simulink model "PV_battery"  (R2020a)
settings: Solver=FixedStepDiscrete  StartTime=0.0  StopTime=20  FixedStep=Tss  RelTol=1e-3
values from neighbouring files (symbols this model uses):
  Ccbattery = 1000e-6    (= 0.001)    [pv_battery.m]
  Ccboost = 3300e-6    (= 0.0033)    [pv_battery.m]
  Ccpv = 100e-6    (= 0.0001)    [pv_battery.m]
  DB_max = 0.95    [pv_battery.m]
  DB_min = 0    [pv_battery.m]
  Delta = 125e-6    (= 0.000125)    [pv_battery.m]
  I_discharge = 22    [pv_battery.m]
  Ki_B1 = 10    [pv_battery.m]
  Ki_B2 = 10    [pv_battery.m]
  Kp_B1 = 0.01    [pv_battery.m]
  Kp_B2 = 0.85    [pv_battery.m]
  LL = 5e-3    (= 0.005)    [pv_battery.m]
  LL1 = 0.5e-3    (= 0.0005)    [pv_battery.m]
  Rcbattery = 1e-4    (= 0.0001)    [pv_battery.m]
  Rcboost = 1e-4    (= 0.0001)    [pv_battery.m]
  Rcpv = 1e-4    (= 0.0001)    [pv_battery.m]
  RL = 0.1    [pv_battery.m]
  RL1 = 0.1    [pv_battery.m]
  Tss = 10e-6    (= 1e-05)    [pv_battery.m]
  Tsspid1 = 5*Tss    (= 5e-05)    [pv_battery.m]
  Tsspid2 = 50*Tss    (= 0.0005)    [pv_battery.m]
  v_bus_ref = 48    [pv_battery.m]
undefined symbols (not defined in the file or in its folder): Ion, Lithium
libraries: powerlib x13, simulink x2, powerlib_meascontrol x2, electricdrivelib x1, re_lib x1
settings Model: Creator=Junaed  LastModifiedBy=Junaed

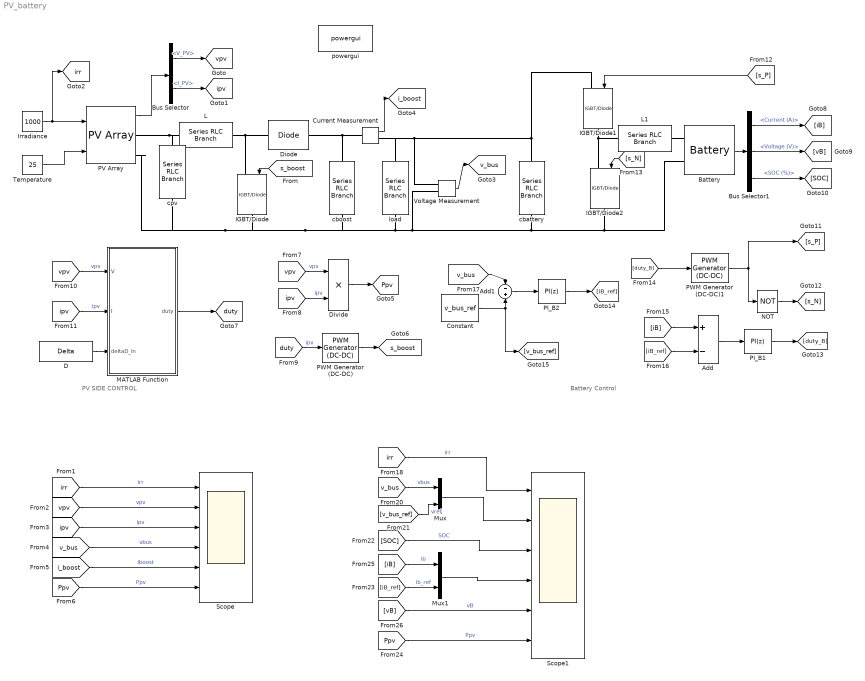
== system PV_battery ==
  note: PV SIDE CONTROL
  note: Battery Control
  Add : Sum  Inputs=+-
  Add1 : Sum  Inputs=-+
  Battery : electricdrivelib/Extra Sources/Battery  BatType=Lithium-Ion  ShowTempParam=off  ThermalPreset=no  ShowAgeParam=off  NomV=Vbat_nom  NomQ=Capacity_nom  SOC=SOC_in  Batt_Tr=1  PresetModel=on  MaxQ=50  MinV=18  FullV=27.9357  Dis_rate=21.7391  R=0.0048  Normal_OP=45.2174  expZone="[25.9293      2.45652]"  current=[6.5 13 32.5]  Units=Time  Tci=20  NomT=20  T2=-30  MaxQ2=4.8  FullV2=7.1  Normal_OP2=5.655  expZone2="[6.58           1]"  Rca=0.6  ti=2000  Dp=0  Neq0=0  Tsim=1e6  Ta1=25  Qeol=5.4*0.9  Reol=0.013333*1.2  Char_age=[2.3478, 3]  Dis_age=[2.3478, 10]  N1=1500  N2=10500  N3=1000  N4=1400  Ta2=45  N5=950
  Bus Selector : BusSelector  OutputSignals=V_PV,I_PV
  Bus Selector1 : BusSelector  OutputSignals=Current (A),Voltage (V),SOC (%)
  Constant : Constant  Value=v_bus_ref
  Current Measurement : powerlib/Measurements/Current Measurement  PhasorSimulation=off  OutputType=Complex  PSBequivalent=0
  D : Constant  Value=Delta
  Diode : powerlib/Power Electronics/Diode  Ron=0.001  Lon=0  Vf=0.8  IC=0  UseSnubber=0  Rs=500  Cs=250e-9  Measurements=off
  Divide : Product  Inputs=**
  IGBT/Diode : powerlib/Power Electronics/IGBT//Diode  Ron=1e-3  Rs=1e5  Cs=inf  Measurements=off
  IGBT/Diode1 : powerlib/Power Electronics/IGBT//Diode  Ron=1e-3  Rs=1e5  Cs=inf  Measurements=off
  IGBT/Diode2 : powerlib/Power Electronics/IGBT//Diode  Ron=1e-3  Rs=1e5  Cs=inf  Measurements=off
  Irradiance : Constant  Value=1000
  L : powerlib/Elements/Series RLC Branch  LConnTagsString=__new0  RConnTagsString=__new0  BranchType=RL  Resistance=RL  Inductance=LL  SetiL0=off  InitialCurrent=0  Capacitance=100e-6  Setx0=off  InitialVoltage=0  Measurements=None
  L1 : powerlib/Elements/Series RLC Branch  LConnTagsString=__new0  RConnTagsString=__new0  BranchType=RL  Resistance=RL1  Inductance=LL1  SetiL0=off  InitialCurrent=0  Capacitance=100e-6  Setx0=off  InitialVoltage=0  Measurements=None
  MATLAB Function : MATLAB Function  TreatAsAtomicUnit=on
  Mux : Mux  Inputs=2
  Mux1 : Mux  Inputs=2
  NOT : Logic  Operator=NOT  IconShape=distinctive  AllPortsSameDT=off  OutDataTypeStr=boolean
  PI_B1 : simulink/Continuous/PID Controller  Controller=PI  Form=Parallel  TimeDomain=Discrete-time  UseExternalTs=off  SampleTime=Tsspid1  IntegratorMethod=Forward Euler  FilterMethod=Forward Euler  ControllerParametersSource=internal  P=Kp_B1  I=Ki_B1  D=0  UseFilter=on  N=100  TunerSelectOption=Transfer Function Based (PID Tuner App)  InitialConditionSource=internal  InitialConditionForIntegrator=0  InitialConditionForFilter=0  DifferentiatorICPrevScaledInput=0  ExternalReset=none  TrackingMode=off  Kt=1  LimitOutput=on  UpperSaturationLimit=DB_max  LowerSaturationLimit=DB_min  LinearizeAsGain=off  AntiWindupMode=none  Kb=1  POutMin=[]  POutMax=[]  IOutMin=[]  IOutMax=[]  DOutMin=[]  DOutMax=[]  NOutMin=[]  NOutMax=[]  SumOutMin=[]  SumOutMax=[]  SaturationOutMin=[]  SaturationOutMax=[]  PParamMin=[]  PParamMax=[]  IParamMin=[]  IParamMax=[]  DParamMin=[]  DParamMax=[]  NParamMin=[]  NParamMax=[]  KbParamMin=[]  KbParamMax=[]  KtParamMin=[]  KtParamMax=[]  KbOutMin=[]  KbOutMax=[]  KtOutMin=[]  KtOutMax=[]  IntegratorOutMin=[]  IntegratorOutMax=[]  FilterOutMin=[]  FilterOutMax=[]  SumI1OutMin=[]  SumI1OutMax=[]  SumI2OutMin=[]  SumI2OutMax=[]  SumI3OutMin=[]  SumI3OutMax=[]  SumI4OutMin=[]  SumI4OutMax=[]  SumDOutMin=[]  SumDOutMax=[]  DifferentiatorOutMin=[]  DifferentiatorOutMax=[]  FilterDiffOutCoefMin=[]  FilterDiffOutCoefMax=[]  ReciprocalOutMin=[]  ReciprocalOutMax=[]  SumDenOutMin=[]  SumDenOutMax=[]  SumNumOutMin=[]  SumNumOutMax=[]  DivideOutMin=[]  DivideOutMax=[]  UdiffTsProdOutMin=[]  UdiffTsProdOutMax=[]  NTsProdOutMin=[]  NTsProdOutMax=[]  UintegralTsProdOutMin=[]  UintegralTsProdOutMax=[]  UngainTsProdOutMin=[]  UngainTsProdOutMax=[]  IntegratorContinuousStateAttributes=''  IntegratorStateMustResolveToSignalObject=off  IntegratorRTWStateStorageClass=Auto  FilterContinuousStateAttributes=''  FilterStateMustResolveToSignalObject=off  FilterRTWStateStorageClass=Auto  ParallelPVariant=InternalParameters  IdealPVariant=Disabled  IVariant=InternalParameters  DVariant=Disabled  IntegratorVariant=Discrete  SatVariant=Enabled  AWVariant=Passthrough  PCopyVariant=Disabled  TRVariant=Disabled  FdbkBlocksVariant=Forward  IdealPFdbkVariant=Disabled  SatFdbkVariant=Disabled  DerivativeFilterVariant=Disabled  NVariant=Disabled  NCopyVariant=Disabled_SignalSpec  FilterICVariant=Disabled  IntegratorICVariant=InternalICs  ExternalResetVariant=Disabled  TRSumVariant=Passthrough  SumFdbkVariant=Disabled  SumVariant=Sum_PI  TsampFilterVariant=InternalTs  TsampNgainVariant=Passthrough  TsampIntegralVariant=Passthrough
  PI_B2 : simulink/Continuous/PID Controller  Controller=PI  Form=Parallel  TimeDomain=Discrete-time  UseExternalTs=off  SampleTime=Tsspid2  IntegratorMethod=Forward Euler  FilterMethod=Forward Euler  ControllerParametersSource=internal  P=Kp_B2  I=Ki_B2  D=0  UseFilter=on  N=100  TunerSelectOption=Transfer Function Based (PID Tuner App)  InitialConditionSource=internal  InitialConditionForIntegrator=0  InitialConditionForFilter=0  DifferentiatorICPrevScaledInput=0  ExternalReset=none  TrackingMode=off  Kt=1  LimitOutput=on  UpperSaturationLimit=I_discharge  LowerSaturationLimit=-I_discharge  LinearizeAsGain=off  AntiWindupMode=none  Kb=1  POutMin=[]  POutMax=[]  IOutMin=[]  IOutMax=[]  DOutMin=[]  DOutMax=[]  NOutMin=[]  NOutMax=[]  SumOutMin=[]  SumOutMax=[]  SaturationOutMin=[]  SaturationOutMax=[]  PParamMin=[]  PParamMax=[]  IParamMin=[]  IParamMax=[]  DParamMin=[]  DParamMax=[]  NParamMin=[]  NParamMax=[]  KbParamMin=[]  KbParamMax=[]  KtParamMin=[]  KtParamMax=[]  KbOutMin=[]  KbOutMax=[]  KtOutMin=[]  KtOutMax=[]  IntegratorOutMin=[]  IntegratorOutMax=[]  FilterOutMin=[]  FilterOutMax=[]  SumI1OutMin=[]  SumI1OutMax=[]  SumI2OutMin=[]  SumI2OutMax=[]  SumI3OutMin=[]  SumI3OutMax=[]  SumI4OutMin=[]  SumI4OutMax=[]  SumDOutMin=[]  SumDOutMax=[]  DifferentiatorOutMin=[]  DifferentiatorOutMax=[]  FilterDiffOutCoefMin=[]  FilterDiffOutCoefMax=[]  ReciprocalOutMin=[]  ReciprocalOutMax=[]  SumDenOutMin=[]  SumDenOutMax=[]  SumNumOutMin=[]  SumNumOutMax=[]  DivideOutMin=[]  DivideOutMax=[]  UdiffTsProdOutMin=[]  UdiffTsProdOutMax=[]  NTsProdOutMin=[]  NTsProdOutMax=[]  UintegralTsProdOutMin=[]  UintegralTsProdOutMax=[]  UngainTsProdOutMin=[]  UngainTsProdOutMax=[]  IntegratorContinuousStateAttributes=''  IntegratorStateMustResolveToSignalObject=off  IntegratorRTWStateStorageClass=Auto  FilterContinuousStateAttributes=''  FilterStateMustResolveToSignalObject=off  FilterRTWStateStorageClass=Auto  ParallelPVariant=InternalParameters  IdealPVariant=Disabled  IVariant=InternalParameters  DVariant=Disabled  IntegratorVariant=Discrete  SatVariant=Enabled  AWVariant=Passthrough  PCopyVariant=Disabled  TRVariant=Disabled  FdbkBlocksVariant=Forward  IdealPFdbkVariant=Disabled  SatFdbkVariant=Disabled  DerivativeFilterVariant=Disabled  NVariant=Disabled  NCopyVariant=Disabled_SignalSpec  FilterICVariant=Disabled  IntegratorICVariant=InternalICs  ExternalResetVariant=Disabled  TRSumVariant=Passthrough  SumFdbkVariant=Disabled  SumVariant=Sum_PI  TsampFilterVariant=InternalTs  TsampNgainVariant=Passthrough  TsampIntegralVariant=Passthrough
  PV Array : re_lib/Solar/PV Array  Npar=Parallel_strings  Nser=series_strings  PlotType=array @ 1000 W/m2 & specified temperatures  S_vec="[ 1000  500  100 ]"  Temp_C_vec="[ 45 25  ]"  ModuleName=1Soltech 1STH-215-P  PlotWhenSelected=off  Pm=213.15  Ncell=60  Voc=36.3  Isc=7.84  Vm=29  Im=7.35  beta_Voc_pc=-0.36099  alpha_Isc_pc=0.102  beta_Voc=-0.13104  alpha_Isc=0.007997  IL=7.8649  I0=2.9259e-10  nI=0.98117  Rsh=313.3991  Rs=0.39383  RobustModel=off  RobustCellTemperature=25  BAL=on  Tc=1e-6  Tfilter=5e-5
  PWM Generator (DC-DC) : powerlib_meascontrol/Pulse & Signal Generators/PWM Generator (DC-DC)  Fsw=fpwm  Ts=Tss
  PWM Generator (DC-DC)1 : powerlib_meascontrol/Pulse & Signal Generators/PWM Generator (DC-DC)  Fsw=fpwm  Ts=Tss
  Scope : Scope  NumInputPorts=6
  Scope1 : Scope  NumInputPorts=6
  Temperature : Constant  Value=25
  Voltage Measurement : powerlib/Measurements/Voltage Measurement  PhasorSimulation=off  OutputType=Complex  PSBequivalent=0
  cbattery : powerlib/Elements/Series RLC Branch  LConnTagsString=__new0  RConnTagsString=__new0  BranchType=RC  Resistance=Rcbattery  Inductance=1e-3  SetiL0=off  InitialCurrent=0  Capacitance=Ccbattery  Setx0=off  InitialVoltage=0  Measurements=None
  cboost : powerlib/Elements/Series RLC Branch  LConnTagsString=__new0  RConnTagsString=__new0  BranchType=RC  Resistance=Rcboost  Inductance=1e-3  SetiL0=off  InitialCurrent=0  Capacitance=Ccboost  Setx0=off  InitialVoltage=0  Measurements=None
  cpv : powerlib/Elements/Series RLC Branch  LConnTagsString=__new0  RConnTagsString=__new0  BranchType=RC  Resistance=Rcpv  Inductance=1e-3  SetiL0=off  InitialCurrent=0  Capacitance=Ccpv  Setx0=off  InitialVoltage=0  Measurements=None
  load : powerlib/Elements/Series RLC Branch  LConnTagsString=__new0  RConnTagsString=__new0  BranchType=R  Resistance=6  Inductance=1e-3  SetiL0=off  InitialCurrent=0  Capacitance=3300e-6  Setx0=off  InitialVoltage=0  Measurements=None
  powergui : powerlib/powergui  Priority=1  SimulationMode=Discrete  SampleTime=Tss  frequency=60  Iterations=50  frequencyindice=0  Pbase=100e6  ErrMax=1e-4  UnitsV=kV  UnitsW=MW  buscounter=0  FunctionMessages=off  echomessages=off  EnableUseOfTLC=off  CurrentSourceSwitches=off  DisableSnubberDevices=off  DisableRonSwitches=off  DisableVfSwitches=off  DisplayEquations=off  AutomaticDiscreteSolvers=off  SolverType=Tustin/Backward Euler (TBE)  Interpol=off  ExternalGateDelay=off  methode=off  Ts=100  x0status=blocks  SPID=on  SwTol=0  HookPort=off  NonlinearTolerance=1e-4  nMaxIteration=100  ContinueOnMaxIteration=off  RestoreLinks=warning  ResistiveCurrentMeasurement=off  Frange=[0:2:500]  Ylog=off  Xlog=on  ShowGrid=off  save=off  variable=ZData  structure=0  ZoomFFT=off  StartTime=0.0  cycles=1  DisplayStyle=1  fundamental=60  FreqAxis=off  MaxFrequency=1000  frequencyindicesteady=1  RmsSteady=1  display=off
  tag scope: Ppv=global, duty=global, i_boost=global, ipv=global, irr=global, s_boost=global, v_bus=global, vpv=global
  wires:
  PV Array/1 -> Bus Selector/1
  Bus Selector/1 -> [vpv]  "<V_PV>"
  Bus Selector/2 -> [ipv]  "<I_PV>"
  Irradiance/1 -> [irr], PV Array/1
  Temperature/1 -> PV Array/2
  [s_boost] -> IGBT/Diode/1
  Voltage Measurement/1 -> [v_bus]
  Current Measurement/1 -> [i_boost]
  [irr] -> Scope/1  "irr"
  [vpv] -> Scope/2  "vpv"
  [ipv] -> Scope/3  "ipv"
  [v_bus] -> Scope/4  "vbus"
  [i_boost] -> Scope/5  "iboost"
  [Ppv] -> Scope/6  "Ppv"
  Divide/1 -> [Ppv]
  [vpv] -> Divide/1  "vpv"
  [ipv] -> Divide/2  "ipv"
  PWM Generator (DC-DC)/1 -> [s_boost]
  [duty] -> PWM Generator (DC-DC)/1  "ipv"
  MATLAB Function/1(duty) -> [duty]
  [vpv] -> MATLAB Function/1(V)  "vpv"
  [ipv] -> MATLAB Function/2(I)  "ipv"
  D/1 -> MATLAB Function/3(deltaD_in)
  Battery/1 -> Bus Selector1/1
  Bus Selector1/1 -> [iB]  "<Current (A)>"
  Bus Selector1/2 -> [vB]  "<Voltage (V)>"
  Bus Selector1/3 -> [SOC]  "<SOC (%)>"
  [s_P] -> IGBT/Diode1/1
  [s_N] -> IGBT/Diode2/1
  PWM Generator (DC-DC)1/1 -> [s_P], NOT/1
  NOT/1 -> [s_N]
  [duty_B] -> PWM Generator (DC-DC)1/1
  PI_B1/1 -> [duty_B]
  Add/1 -> PI_B1/1
  [iB] -> Add/1
  [iB_ref] -> Add/2
  PI_B2/1 -> [iB_ref]
  [v_bus] -> Add1/1
  Add1/1 -> PI_B2/1
  [Ppv] -> Scope1/6  "Ppv"
  [irr] -> Scope1/1  "irr"
  Mux/1 -> Scope1/2
  [v_bus] -> Mux/1  "vbus"
  [v_bus_ref] -> Mux/2  "vref"
  [SOC] -> Scope1/3  "SOC"
  [iB] -> Mux1/1  "ib"
  Mux1/1 -> Scope1/4
  [iB_ref] -> Mux1/2  "ib_ref"
  [vB] -> Scope1/5  "vB"
  Constant/1 -> [v_bus_ref], Add1/2
  connections:
  PV Array/RConn1 -- L/RConn1 -- cpv/LConn1
  Battery/LConn2 -- IGBT/Diode2/RConn1 -- cboost/RConn1 -- IGBT/Diode/RConn1 -- PV Array/RConn2 -- cpv/RConn1 -- load/RConn1 -- Voltage Measurement/LConn2 -- cbattery/RConn1
  L/LConn1 -- Diode/LConn1 -- IGBT/Diode/LConn1
  cboost/LConn1 -- Current Measurement/LConn1 -- Diode/RConn1
  L1/LConn1 -- Battery/LConn1
  L1/RConn1 -- IGBT/Diode2/LConn1 -- IGBT/Diode1/RConn1
  IGBT/Diode1/LConn1 -- load/LConn1 -- Current Measurement/RConn1 -- Voltage Measurement/LConn1 -- cbattery/LConn1

== matlab function PV_battery/MATLAB Function ==
  data: V input; duty output; I input; deltaD_in input
function duty = MPPT_Control(V,I,deltaD_in)

duty_init = 0.05;
duty_min = 0;
duty_max=0.75;

persistent Vold Pold duty_old ;

if isempty(Vold)
    Vold = 0;
    Pold = 0;
    duty_old = duty_init;
end
P=V*I;
dV=V-Vold;
dP=P-Pold;
duty=duty_old;
deltaD=deltaD_in;

if dP~=0
    if dP<0
        if dV<0
            duty = duty_old-deltaD;
        else
            duty = duty_old+deltaD;
        end
    else
        if dV<0
            duty = duty_old+deltaD;
        else
            duty = duty_old-deltaD;
        end
    end
end
if duty >=duty_max
    duty=duty_max;
elseif duty< duty_min
    duty=duty_min;
end
duty_old = duty;
Vold=V;
Pold=P;
end
